simulink subsystem "s2e_to_3s"  (R2022b)
settings: Solver=VariableStepAuto  StartTime=0.0  StopTime=10.0  RelTol=1e-3
settings Model: Creator=jack  LastModifiedBy=jack

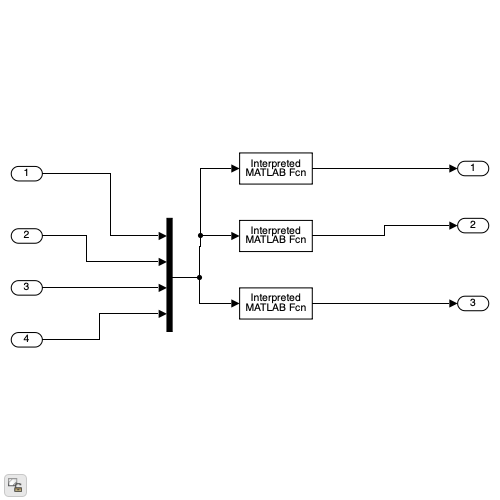
[thumbnail: Simulink's stored preview of the top-level diagram]
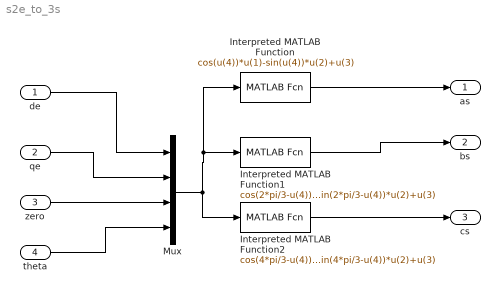
== system s2e_to_3s ==
  de : Inport
  qe : Inport  Port=2
  zero : Inport  Port=3
  theta : Inport  Port=4
  Interpreted MATLAB Function : MATLABFcn  MATLABFcn=cos(u(4))*u(1)-sin(u(4))*u(2)+u(3)
  Interpreted MATLAB Function1 : MATLABFcn  MATLABFcn=cos(2*pi/3-u(4))*u(1)+sin(2*pi/3-u(4))*u(2)+u(3)
  Interpreted MATLAB Function2 : MATLABFcn  MATLABFcn=cos(4*pi/3-u(4))*u(1)+sin(4*pi/3-u(4))*u(2)+u(3)
  Mux : Mux
  as : Outport
  bs : Outport  Port=2
  cs : Outport  Port=3
  wires:
  theta/1 -> Mux/4
  Interpreted MATLAB Function/1 -> as/1
  qe/1 -> Mux/2
  de/1 -> Mux/1
  Interpreted MATLAB Function1/1 -> bs/1
  Mux/1 -> Interpreted MATLAB Function2/1, Interpreted MATLAB Function1/1, Interpreted MATLAB Function/1
  zero/1 -> Mux/3
  Interpreted MATLAB Function2/1 -> cs/1
